simulink model "SingleStreamSSRwithPL"  (R2020a)
settings: Solver=VariableStepAuto  StartTime=0.0  StopTime=inf  RelTol=1e-3
PreLoadFcn:
  | xmcCheckSlxPath(bdroot)
  | SSR4_init
InitFcn:
  | xmcCheckSlxPath(bdroot)
  | SSR4_init;
undefined symbols (not defined in the file): c, FIR_MultiKernel_cin, FIR_MultiKernel_cincout, FIR_MultiKernel_cout, FramesPerVector, S, SHIFT_ACC, SingleStream, T, Taps, ValidDelay, VectorSize, xc7vx485tffg1157
libraries: xbsIndex_r4 x49, ModelComposer x41, simulink x25, dspsrcs4 x1
(part 1 of 3)
settings Model: Creator=oliviert  LastModifiedBy=viswanad

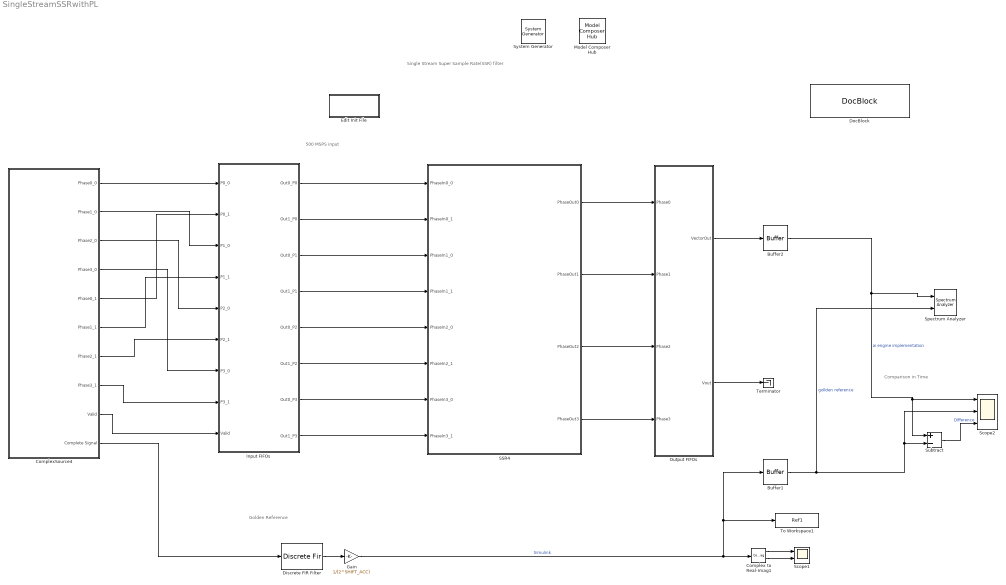
== system SingleStreamSSRwithPL ==
  note: Golden Reference
  note: Single Stream Super Sample Rate(SSR) filter
  note: Comparison in Time
  note: 500 MSPS input
  " System Generator" : xbsIndex_r4/ System Generator  Tag=genX  xilinxfamily=versalaicore  part=xcvc1902  speed=-2MP-e-S  package=vsva2197  synthesis_tool=Vivado  clock_wrapper=Clock Enables  directory=./netlist  proj_type=Vivado  Synth_file=Vivado Synthesis Defaults  Impl_file=Vivado Implementation Defaults  testbench=off  simulink_period=1  sysclk_period=10  dcm_input_clock_period=10  incr_netlist=off  trim_vbits=Everywhere in SubSystem  dbl_ovrd=According to Block Masks  core_generation=According to Block Masks  run_coregen=off  deprecated_control=off  eval_field=0  block_type=sysgen
  Buffer1 : Buffer  N=16  OutputFrames=off
  Buffer2 : Buffer  N=16  OutputFrames=off
  Complex to Real-Imag1 : ComplexToRealImag
  ComplexSource4 : Subsystem  mask{s=0}
      mask prompts: s "Seed"
  Discrete FIR Filter : DiscreteFir  Coefficients=Taps  InputProcessing=Columns as channels (frame based)
  DocBlock : simulink/Model-Wide Utilities/DocBlock  DocumentType=Text  mask(DocBlock){}
      content=|
      | ///////////////////////////////////////////////////////////////////////////
      | // Copyright 2020 Xilinx
      | //
      | // Licensed under the Apache License, Version 2.0 (the "License");
      | // you may not use this file except in compliance with the License.
      | // You may obtain a copy of the License at
      | //
      | // http://www.apache.org/licenses/LICENSE-2.0
      | //
      | // Unless required by applicable law or agreed to in writing, software
      | // distributed under the License is distributed on an "AS IS" BASIS,
      | // WITHOUT WARRANTIES OR CONDITIONS OF ANY KIND, either express or implied.
      | // See the License for the specific language governing permissions and
      | // limitations under the License.
      | ///////////////////////////////////////////////////////////////////////////
      mask Display:
      | xmcDrawBlockIcon();
      | disp(['{\fontsize{10pt}(c) Copyright 2020' ' Xilinx, Inc.}\newline \newline '],'texmode','on');
      | disp('{\fontsize{10pt}Licensed under the Apache License 2.0}','texmode','on');
      | disp('\newline \newline \newline{\fontsize{10pt}Double Click for Copyright Notice}','texmode','on');
  Edit Init File : Subsystem
      settings: OpenFcn=edit('SSR4_init.m');
  Gain : Gain  Gain=1/(2^SHIFT_ACC)
  Input FIFOs : Subsystem
  Model Composer Hub : ModelComposer/Model Composer Hub  CodeGeneration=off  SubsystemName=SSR4  TargetDirectory=./code  ExportType=AI Engines  IpVendor=xilinx.com  IpLibrary=hls  IpVersion=1.0  IpHWLanguage=Verilog  AieCompilerOptions={}  CreateTestbench=on  TestbenchStackSize=10  RunAieSim=on  AieSimTimeout=5000  RunAieSimProfiling=off  LaunchVitisAnalyzer=on  PlotOutput=off  RunX86Sim=off  X86SimTimeout=10  GenHwImage=off  PlatformType=Not Specified  ProjDevice=xc7vx485tffg1157-1  ProjDevicePart=xc7vx485tffg1157-1  SamplePeriod=-1  ClockFrequency=200  DataPathParallelism=1
  Output FIFOs : Subsystem
  SSR4 : Subsystem
  Scope1 : Scope  NumInputPorts=2
  Scope2 : Scope  NumInputPorts=3
  Spectrum Analyzer : SpectrumAnalyzer  NumInputPorts=2
  Subtract : Sum  Inputs=+-
  Terminator : Terminator
  To Workspace1 : ToWorkspace  VariableName=Ref1  SampleTime=-1
      settings: Save2DSignal=2-D array (concatenate along first dimension)
  wires:
  ComplexSource4/10(Complete Signal) -> Discrete FIR Filter/1
  Discrete FIR Filter/1 -> Gain/1
  ComplexSource4/2(Phase1_0) -> Input FIFOs/3(P1_0)
  ComplexSource4/3(Phase2_0) -> Input FIFOs/5(P2_0)
  ComplexSource4/4(Phase3_0) -> Input FIFOs/7(P3_0)
  ComplexSource4/9(Valid) -> Input FIFOs/9(Valid)
  ComplexSource4/5(Phase0_1) -> Input FIFOs/2(P0_1)
  ComplexSource4/6(Phase1_1) -> Input FIFOs/4(P1_1)
  ComplexSource4/7(Phase2_1) -> Input FIFOs/6(P2_1)
  ComplexSource4/8(Phase3_1) -> Input FIFOs/8(P3_1)
  ComplexSource4/1(Phase0_0) -> Input FIFOs/1(P0_0)
  Input FIFOs/1(Out0_P0) -> SSR4/1(PhaseIn0_0)
  Input FIFOs/2(Out1_P0) -> SSR4/2(PhaseIn0_1)
  Input FIFOs/3(Out0_P1) -> SSR4/3(PhaseIn1_0)
  Input FIFOs/4(Out1_P1) -> SSR4/4(PhaseIn1_1)
  Input FIFOs/5(Out0_P2) -> SSR4/5(PhaseIn2_0)
  Input FIFOs/6(Out1_P2) -> SSR4/6(PhaseIn2_1)
  Input FIFOs/7(Out0_P3) -> SSR4/7(PhaseIn3_0)
  Input FIFOs/8(Out1_P3) -> SSR4/8(PhaseIn3_1)
  Subtract/1 -> Scope2/3  "Difference"
  Complex to Real-Imag1/2 -> Scope1/2
  SSR4/1(PhaseOut0) -> Output FIFOs/1(Phase0)
  Complex to Real-Imag1/1 -> Scope1/1
  Gain/1 -> Buffer1/1, To Workspace1/1, Complex to Real-Imag1/1  "Simulink"
  Buffer1/1 -> Spectrum Analyzer/2, Subtract/2, Scope2/2  "gollden reference"
  Output FIFOs/1(VectorOut) -> Buffer2/1
  SSR4/2(PhaseOut1) -> Output FIFOs/2(Phase1)
  SSR4/3(PhaseOut2) -> Output FIFOs/3(Phase2)
  SSR4/4(PhaseOut3) -> Output FIFOs/4(Phase3)
  Buffer2/1 -> Subtract/1, Scope2/1, Spectrum Analyzer/1  "ai engine implementation"
  Output FIFOs/2(Vout) -> Terminator/1

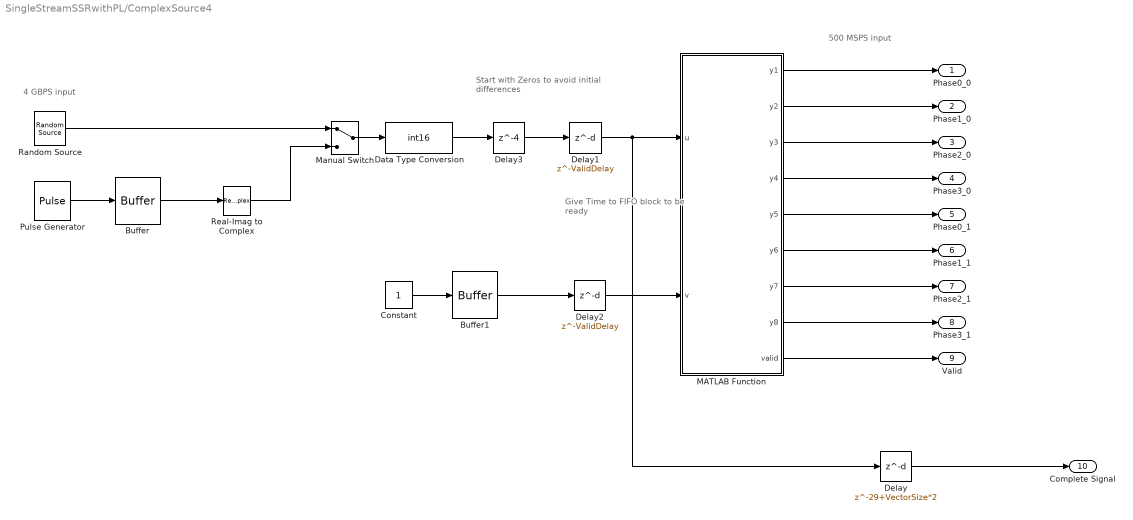
== system SingleStreamSSRwithPL/ComplexSource4 ==
  note: Give Time to
      | FIFO block
      | to be ready
  note: Start with Zeros
      | to avoid
      | initial differences
  note: 4 GBPS input
  note: 500 MSPS input
  Buffer : Buffer  N=VectorSize  OutputFrames=off
  Buffer1 : Buffer  N=FramesPerVector  OutputFrames=off
  Constant : Constant  SampleTime=1
  Data Type Conversion : DataTypeConversion  OutDataTypeStr=int16
  Delay : Delay  DelayLength=29+VectorSize*2  InputProcessing=Columns as channels (frame based)
  Delay1 : Delay  DelayLength=ValidDelay
  Delay2 : Delay  DelayLength=ValidDelay
  Delay3 : Delay  DelayLength=4
  MATLAB Function : MATLAB Function  TreatAsAtomicUnit=on
  Manual Switch : ManualSwitch
  Pulse Generator : DiscretePulseGenerator  Amplitude=20000  Period=32 + 40*5  PhaseDelay=32  SampleTime=1/T
  Random Source : dspsrcs4/Random Source  SrcType=Uniform  NormMethod=Ziggurat  CltLength=12  MinVal=-20000  MaxVal=20000  MeanVal=0  VarVal=1  RepMode=Specify seed  rawSeed=s  IsInherit=off  SampMode=Discrete  SampTime=1/T  SampFrame=VectorSize  DataType=Double  OutComplex=Complex  OutputFrames=off
  Real-Imag to Complex : RealImagToComplex  Input=Real
  Phase0_0 : Outport
  Phase1_0 : Outport  Port=2
  Phase2_0 : Outport  Port=3
  Phase3_0 : Outport  Port=4
  Phase0_1 : Outport  Port=5
  Phase1_1 : Outport  Port=6
  Phase2_1 : Outport  Port=7
  Phase3_1 : Outport  Port=8
  Valid : Outport  Port=9
  Complete Signal : Outport  Port=10
  wires:
  MATLAB Function/1(y1) -> Phase0_0/1
  MATLAB Function/2(y2) -> Phase1_0/1
  MATLAB Function/3(y3) -> Phase2_0/1
  MATLAB Function/4(y4) -> Phase3_0/1
  Real-Imag to Complex/1 -> Manual Switch/2
  Pulse Generator/1 -> Buffer/1
  Delay/1 -> Complete Signal/1
  Buffer/1 -> Real-Imag to Complex/1
  Manual Switch/1 -> Data Type Conversion/1
  MATLAB Function/9(valid) -> Valid/1
  MATLAB Function/8(y8) -> Phase3_1/1
  MATLAB Function/7(y7) -> Phase2_1/1
  MATLAB Function/6(y6) -> Phase1_1/1
  MATLAB Function/5(y5) -> Phase0_1/1
  Random Source/1 -> Manual Switch/1
  Delay1/1 -> Delay/1, MATLAB Function/1(u)
  Delay2/1 -> MATLAB Function/2(v)
  Constant/1 -> Buffer1/1
  Buffer1/1 -> Delay2/1
  Data Type Conversion/1 -> Delay3/1
  Delay3/1 -> Delay1/1

== system SingleStreamSSRwithPL/Edit Init File ==

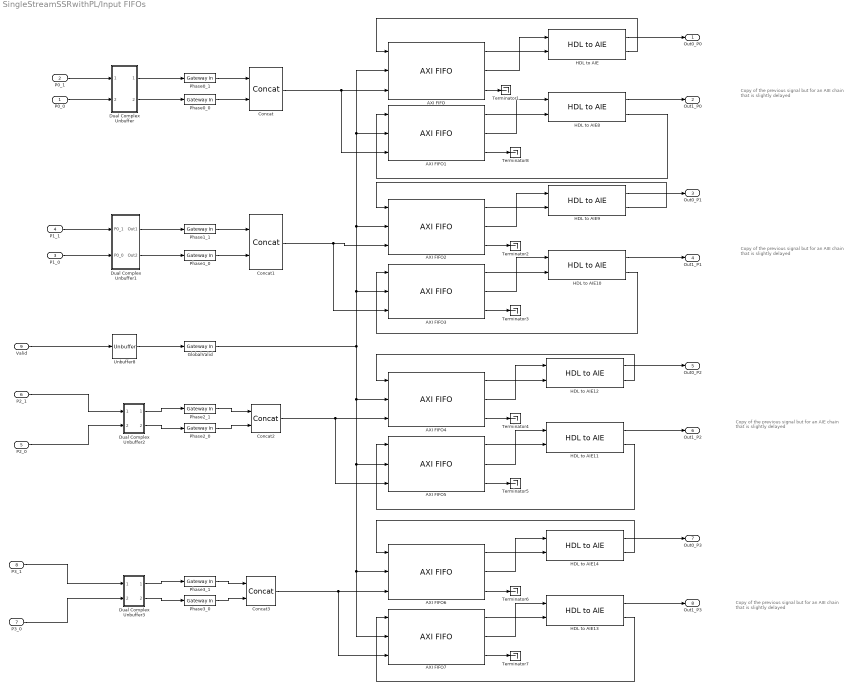
== system SingleStreamSSRwithPL/Input FIFOs ==
  note: Copy of the previous signal
      | but for an AIE chain that is slightly
      | delayed
  note: Copy of the previous signal
      | but for an AIE chain that is slightly
      | delayed
  note: Copy of the previous signal
      | but for an AIE chain that is slightly
      | delayed
  note: Copy of the previous signal
      | but for an AIE chain that is slightly
      | delayed
  P0_0 : Inport
  P0_1 : Inport  Port=2
  P1_0 : Inport  Port=3
  P1_1 : Inport  Port=4
  P2_0 : Inport  Port=5
  P2_1 : Inport  Port=6
  P3_0 : Inport  Port=7
  P3_1 : Inport  Port=8
  Valid : Inport  Port=9
  AXI FIFO{,1..7} (8 alike) : xbsIndex_r4/AXI FIFO  input_depth_axis=512  actual_fifo_depth_label=514  enable_tdata=on  enable_tdest=off  enable_tstrb=off  enable_tready=on  enable_tid=off  enable_tuser=off  enable_tkeep=off  enable_tlast=off  has_aresetn=off  enable_data_counts_axis=off  fifo_implementation_type_axis=Common Clock Block RAM  trim_axipin_name=on  programmable_full_type_axis=Full  full_threshold_assert_value_axis=0  programmable_empty_type_axis=Empty  empty_threshold_assert_value_axis=1022  underflow_flag_axi=0  underflow_sense_axi=Active High  overflow_flag_axi=0  overflow_sense_axi=Active High  simulation_type=fast_sim  block_type=axi_fifo
  Concat{,1..3} (4 alike) : xbsIndex_r4/Concat  num_inputs=2  dbl_ovrd=off  block_type=concat
  Dual Complex Unbuffer : Subsystem
  Dual Complex Unbuffer1 : Subsystem
  Dual Complex Unbuffer2 : Subsystem
  Dual Complex Unbuffer3 : Subsystem
  GlobalValid : xbsIndex_r4/Gateway In  gui_display_data_type=Boolean  arith_type=Boolean  n_bits=16  bin_pt=14  preci_type=Single  exp_width=8  frac_width=24  rows=1  columns=1  quantization="Round  (unbiased: +/- Inf)"  overflow=Saturate  period=1  UseAsADC=off  ADCChannel='1'  interface=None  automatic_assignment=on  address_offset=hex2dec('00')  intf_name=''  intf_description=''  default_value=0  timing_constraint=None  locs_specified=off  LOCs={}  io_standard={}  inherit_from_input=off  hdl_port=on  dbl_ovrd=off  block_type=gatewayin
  HDL to AIE{,8..14} (8 alike) : ModelComposer/HDL to AIE  OutDataType=int16 (c)  OutSampleTime=4/T  SamplesPerFrame=4  TreadySampleTime=1
  Phase0_0 : xbsIndex_r4/Gateway In  gui_display_data_type=Fixed-point  arith_type=Unsigned  n_bits=32  bin_pt=0  preci_type=Single  exp_width=8  frac_width=24  rows=1  columns=1  quantization="Round  (unbiased: +/- Inf)"  overflow=Saturate  period=1  UseAsADC=off  ADCChannel='1'  interface=None  automatic_assignment=on  address_offset=hex2dec('00')  intf_name=''  intf_description=''  default_value=0  timing_constraint=None  locs_specified=off  LOCs={}  io_standard={}  inherit_from_input=off  hdl_port=on  dbl_ovrd=off  block_type=gatewayin
  Phase0_1 : xbsIndex_r4/Gateway In  gui_display_data_type=Fixed-point  arith_type=Unsigned  n_bits=32  bin_pt=0  preci_type=Single  exp_width=8  frac_width=24  rows=1  columns=1  quantization="Round  (unbiased: +/- Inf)"  overflow=Saturate  period=1  UseAsADC=off  ADCChannel='1'  interface=None  automatic_assignment=on  address_offset=hex2dec('00')  intf_name=''  intf_description=''  default_value=0  timing_constraint=None  locs_specified=off  LOCs={}  io_standard={}  inherit_from_input=off  hdl_port=on  dbl_ovrd=off  block_type=gatewayin
  Phase1_0 : xbsIndex_r4/Gateway In  gui_display_data_type=Fixed-point  arith_type=Unsigned  n_bits=32  bin_pt=0  preci_type=Single  exp_width=8  frac_width=24  rows=1  columns=1  quantization="Round  (unbiased: +/- Inf)"  overflow=Saturate  period=1  UseAsADC=off  ADCChannel='1'  interface=None  automatic_assignment=on  address_offset=hex2dec('00')  intf_name=''  intf_description=''  default_value=0  timing_constraint=None  locs_specified=off  LOCs={}  io_standard={}  inherit_from_input=off  hdl_port=on  dbl_ovrd=off  block_type=gatewayin
  Phase1_1 : xbsIndex_r4/Gateway In  gui_display_data_type=Fixed-point  arith_type=Unsigned  n_bits=32  bin_pt=0  preci_type=Single  exp_width=8  frac_width=24  rows=1  columns=1  quantization="Round  (unbiased: +/- Inf)"  overflow=Saturate  period=1  UseAsADC=off  ADCChannel='1'  interface=None  automatic_assignment=on  address_offset=hex2dec('00')  intf_name=''  intf_description=''  default_value=0  timing_constraint=None  locs_specified=off  LOCs={}  io_standard={}  inherit_from_input=off  hdl_port=on  dbl_ovrd=off  block_type=gatewayin
  Phase2_0 : xbsIndex_r4/Gateway In  gui_display_data_type=Fixed-point  arith_type=Unsigned  n_bits=32  bin_pt=0  preci_type=Single  exp_width=8  frac_width=24  rows=1  columns=1  quantization="Round  (unbiased: +/- Inf)"  overflow=Saturate  period=1  UseAsADC=off  ADCChannel='1'  interface=None  automatic_assignment=on  address_offset=hex2dec('00')  intf_name=''  intf_description=''  default_value=0  timing_constraint=None  locs_specified=off  LOCs={}  io_standard={}  inherit_from_input=off  hdl_port=on  dbl_ovrd=off  block_type=gatewayin
  Phase2_1 : xbsIndex_r4/Gateway In  gui_display_data_type=Fixed-point  arith_type=Unsigned  n_bits=32  bin_pt=0  preci_type=Single  exp_width=8  frac_width=24  rows=1  columns=1  quantization="Round  (unbiased: +/- Inf)"  overflow=Saturate  period=1  UseAsADC=off  ADCChannel='1'  interface=None  automatic_assignment=on  address_offset=hex2dec('00')  intf_name=''  intf_description=''  default_value=0  timing_constraint=None  locs_specified=off  LOCs={}  io_standard={}  inherit_from_input=off  hdl_port=on  dbl_ovrd=off  block_type=gatewayin
  Phase3_0 : xbsIndex_r4/Gateway In  gui_display_data_type=Fixed-point  arith_type=Unsigned  n_bits=32  bin_pt=0  preci_type=Single  exp_width=8  frac_width=24  rows=1  columns=1  quantization="Round  (unbiased: +/- Inf)"  overflow=Saturate  period=1  UseAsADC=off  ADCChannel='1'  interface=None  automatic_assignment=on  address_offset=hex2dec('00')  intf_name=''  intf_description=''  default_value=0  timing_constraint=None  locs_specified=off  LOCs={}  io_standard={}  inherit_from_input=off  hdl_port=on  dbl_ovrd=off  block_type=gatewayin
  Phase3_1 : xbsIndex_r4/Gateway In  gui_display_data_type=Fixed-point  arith_type=Unsigned  n_bits=32  bin_pt=0  preci_type=Single  exp_width=8  frac_width=24  rows=1  columns=1  quantization="Round  (unbiased: +/- Inf)"  overflow=Saturate  period=1  UseAsADC=off  ADCChannel='1'  interface=None  automatic_assignment=on  address_offset=hex2dec('00')  intf_name=''  intf_description=''  default_value=0  timing_constraint=None  locs_specified=off  LOCs={}  io_standard={}  inherit_from_input=off  hdl_port=on  dbl_ovrd=off  block_type=gatewayin
  Terminator{1..8} (8 alike) : Terminator
  Unbuffer8 : Unbuffer
  Out0_P0 : Outport
  Out1_P0 : Outport  Port=2
  Out0_P1 : Outport  Port=3
  Out1_P1 : Outport  Port=4
  Out0_P2 : Outport  Port=5
  Out1_P2 : Outport  Port=6
  Out0_P3 : Outport  Port=7
  Out1_P3 : Outport  Port=8
  wires:
  P0_0/1 -> Dual Complex Unbuffer/2(P0_0)
  Valid/1 -> Unbuffer8/1
  GlobalValid/1 -> AXI FIFO4/2, AXI FIFO6/2, AXI FIFO7/2, AXI FIFO5/2, AXI FIFO3/2, AXI FIFO2/2, AXI FIFO1/2, AXI FIFO/2
  Phase2_1/1 -> Concat2/1
  Phase2_0/1 -> Concat2/2
  Phase3_1/1 -> Concat3/1
  Phase3_0/1 -> Concat3/2
  Phase1_0/1 -> Concat1/2
  Phase1_1/1 -> Concat1/1
  Phase0_1/1 -> Concat/1
  Phase0_0/1 -> Concat/2
  Concat/1 -> AXI FIFO1/3, AXI FIFO/3
  AXI FIFO1/3 -> Terminator8/1
  Concat1/1 -> AXI FIFO3/3, AXI FIFO2/3
  AXI FIFO2/3 -> Terminator2/1
  AXI FIFO3/3 -> Terminator3/1
  AXI FIFO5/3 -> Terminator5/1
  AXI FIFO4/3 -> Terminator4/1
  Concat2/1 -> AXI FIFO5/3, AXI FIFO4/3
  AXI FIFO6/3 -> Terminator6/1
  AXI FIFO7/3 -> Terminator7/1
  Concat3/1 -> AXI FIFO7/3, AXI FIFO6/3
  AXI FIFO/1 -> HDL to AIE/2
  AXI FIFO/2 -> HDL to AIE/1
  HDL to AIE/1 -> Out0_P0/1
  AXI FIFO1/1 -> HDL to AIE8/2
  AXI FIFO1/2 -> HDL to AIE8/1
  HDL to AIE8/1 -> Out1_P0/1
  HDL to AIE8/2 -> AXI FIFO1/1
  AXI FIFO2/1 -> HDL to AIE9/2
  AXI FIFO3/1 -> HDL to AIE10/2
  AXI FIFO2/2 -> HDL to AIE9/1
  AXI FIFO3/2 -> HDL to AIE10/1
  HDL to AIE10/2 -> AXI FIFO3/1
  HDL to AIE9/1 -> Out0_P1/1
  HDL to AIE10/1 -> Out1_P1/1
  HDL to AIE9/2 -> AXI FIFO2/1
  AXI FIFO4/1 -> HDL to AIE12/2
  AXI FIFO4/2 -> HDL to AIE12/1
  HDL to AIE12/1 -> Out0_P2/1
  HDL to AIE11/1 -> Out1_P2/1
  HDL to AIE12/2 -> AXI FIFO4/1
  AXI FIFO5/1 -> HDL to AIE11/2
  AXI FIFO5/2 -> HDL to AIE11/1
  HDL to AIE11/2 -> AXI FIFO5/1
  AXI FIFO6/1 -> HDL to AIE14/2
  HDL to AIE14/1 -> Out0_P3/1
  HDL to AIE13/1 -> Out1_P3/1
  AXI FIFO6/2 -> HDL to AIE14/1
  AXI FIFO7/1 -> HDL to AIE13/2
  AXI FIFO7/2 -> HDL to AIE13/1
  HDL to AIE14/2 -> AXI FIFO6/1
  HDL to AIE13/2 -> AXI FIFO7/1
  Unbuffer8/1 -> GlobalValid/1
  Dual Complex Unbuffer/1(Out1) -> Phase0_1/1
  Dual Complex Unbuffer/2(Out2) -> Phase0_0/1
  Dual Complex Unbuffer1/1(Out1) -> Phase1_1/1
  Dual Complex Unbuffer1/2(Out2) -> Phase1_0/1
  P1_1/1 -> Dual Complex Unbuffer1/1(P0_1)
  P1_0/1 -> Dual Complex Unbuffer1/2(P0_0)
  Dual Complex Unbuffer2/1(Out1) -> Phase2_1/1
  Dual Complex Unbuffer2/2(Out2) -> Phase2_0/1
  P2_1/1 -> Dual Complex Unbuffer2/1(P0_1)
  P2_0/1 -> Dual Complex Unbuffer2/2(P0_0)
  Dual Complex Unbuffer3/1(Out1) -> Phase3_1/1
  Dual Complex Unbuffer3/2(Out2) -> Phase3_0/1
  P3_1/1 -> Dual Complex Unbuffer3/1(P0_1)
  P3_0/1 -> Dual Complex Unbuffer3/2(P0_0)
  P0_1/1 -> Dual Complex Unbuffer/1(P0_1)
  HDL to AIE/2 -> AXI FIFO/1
  AXI FIFO/3 -> Terminator1/1

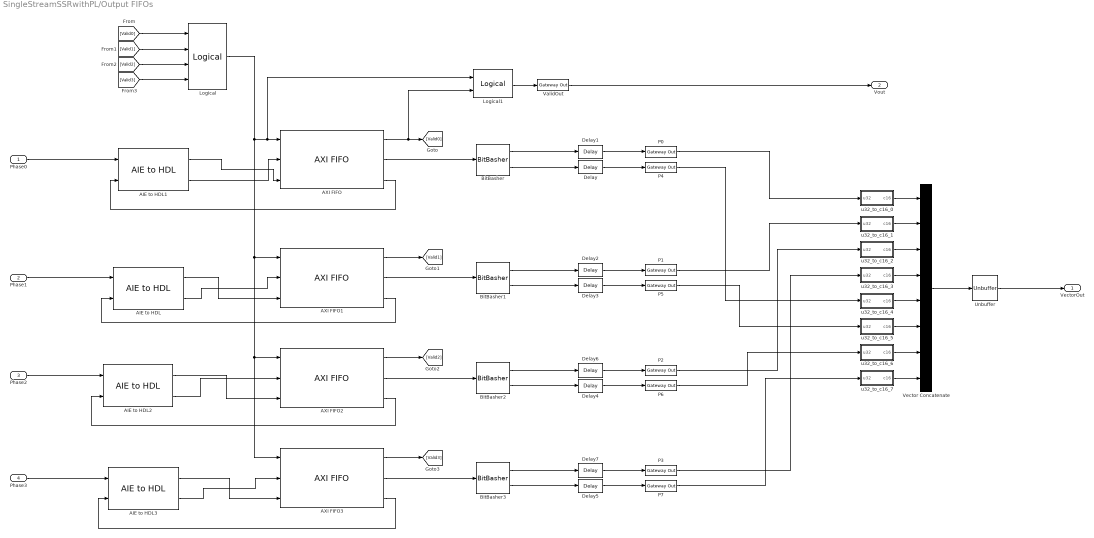
== system SingleStreamSSRwithPL/Output FIFOs ==
  Phase0 : Inport
  Phase1 : Inport  Port=2
  Phase2 : Inport  Port=3
  Phase3 : Inport  Port=4
  AIE to HDL{,1..3} (4 alike) : ModelComposer/AIE to HDL  OutDataType=ufix64  OutSampleTime=1
  AXI FIFO{,1..3} (4 alike) : xbsIndex_r4/AXI FIFO  input_depth_axis=512  actual_fifo_depth_label=514  enable_tdata=on  enable_tdest=off  enable_tstrb=off  enable_tready=on  enable_tid=off  enable_tuser=off  enable_tkeep=off  enable_tlast=off  has_aresetn=off  enable_data_counts_axis=off  fifo_implementation_type_axis=Common Clock Block RAM  trim_axipin_name=on  programmable_full_type_axis=Full  full_threshold_assert_value_axis=0  programmable_empty_type_axis=Empty  empty_threshold_assert_value_axis=1022  underflow_flag_axi=0  underflow_sense_axi=Active High  overflow_flag_axi=0  overflow_sense_axi=Active High  simulation_type=fast_sim  block_type=axi_fifo
  BitBasher : xbsIndex_r4/BitBasher  bitexpr=|  display_expr=off  sr_1=lo  arith_type1=Unsigned  bin_pt1=0  sr_2=hi  arith_type2=Unsigned  bin_pt2=0  sr_3=3  arith_type3=Unsigned  bin_pt3=0  sr_4=4  arith_type4=Unsigned  bin_pt4=0  dbl_ovrd=off  block_type=bitbasher
      | lo={in[31:0]}
      | hi={in[63:32]}
  BitBasher1 : xbsIndex_r4/BitBasher  bitexpr=|  display_expr=off  sr_1=lo  arith_type1=Unsigned  bin_pt1=0  sr_2=hi  arith_type2=Unsigned  bin_pt2=0  sr_3=3  arith_type3=Unsigned  bin_pt3=0  sr_4=4  arith_type4=Unsigned  bin_pt4=0  dbl_ovrd=off  block_type=bitbasher
      | lo={in[31:0]}
      | hi={in[63:32]}
  BitBasher2 : xbsIndex_r4/BitBasher  bitexpr=|  display_expr=off  sr_1=lo  arith_type1=Unsigned  bin_pt1=0  sr_2=hi  arith_type2=Unsigned  bin_pt2=0  sr_3=3  arith_type3=Unsigned  bin_pt3=0  sr_4=4  arith_type4=Unsigned  bin_pt4=0  dbl_ovrd=off  block_type=bitbasher
      | lo={in[31:0]}
      | hi={in[63:32]}
  BitBasher3 : xbsIndex_r4/BitBasher  bitexpr=|  display_expr=off  sr_1=lo  arith_type1=Unsigned  bin_pt1=0  sr_2=hi  arith_type2=Unsigned  bin_pt2=0  sr_3=3  arith_type3=Unsigned  bin_pt3=0  sr_4=4  arith_type4=Unsigned  bin_pt4=0  dbl_ovrd=off  block_type=bitbasher
      | lo={in[31:0]}
      | hi={in[63:32]}
  Delay{,1..7} (8 alike) : xbsIndex_r4/Delay  rst=off  infoeditControl=Selection of Reset will increase slice count due to use of real FFs and instead of SRLs  en=off  latency=1  reg_retiming=off  dbl_ovrd=off  block_type=delay
  Logical : xbsIndex_r4/Logical  logical_function=AND  inputs=4  en=off  latency=0  precision=Full  arith_type=Unsigned  n_bits=16  bin_pt=0  align_bp=on  dbl_ovrd=off  block_type=logical
  Logical1 : xbsIndex_r4/Logical  logical_function=AND  inputs=2  en=off  latency=1  precision=Full  arith_type=Unsigned  n_bits=16  bin_pt=0  align_bp=on  dbl_ovrd=off  block_type=logical
  P{0..7} (8 alike) : xbsIndex_r4/Gateway Out  inherit_from_input=on  hdl_port=on  rows=1  columns=1  UseAsDAC=off  DACChannel='1'  interface=None  automatic_assignment=on  address_offset=hex2dec('00')  intf_name=''  intf_description=''  timing_constraint=None  locs_specified=off  LOCs={}  io_standard={}  block_type=gatewayout
  Unbuffer : Unbuffer
  ValidOut : xbsIndex_r4/Gateway Out  inherit_from_input=off  hdl_port=on  rows=1  columns=1  UseAsDAC=off  DACChannel='1'  interface=None  automatic_assignment=on  address_offset=hex2dec('00')  intf_name=''  intf_description=''  timing_constraint=None  locs_specified=off  LOCs={}  io_standard={}  block_type=gatewayout
  Vector Concatenate : Concatenate  NumInputs=8
  u32_to_c16_0 : Subsystem
  u32_to_c16_1 : Subsystem
  u32_to_c16_2 : Subsystem
  u32_to_c16_3 : Subsystem
  u32_to_c16_4 : Subsystem
  u32_to_c16_5 : Subsystem
  u32_to_c16_6 : Subsystem
  u32_to_c16_7 : Subsystem
  VectorOut : Outport
  Vout : Outport  Port=2
  wires:
  Phase0/1 -> AIE to HDL1/1
  AXI FIFO/3 -> AIE to HDL1/2
  AXI FIFO1/3 -> AIE to HDL/2
  Phase1/1 -> AIE to HDL/1
  Phase2/1 -> AIE to HDL2/1
  AXI FIFO2/3 -> AIE to HDL2/2
  AXI FIFO3/3 -> AIE to HDL3/2
  Phase3/1 -> AIE to HDL3/1
  Logical/1 -> Logical1/1, AXI FIFO/1, AXI FIFO1/1, AXI FIFO2/1, AXI FIFO3/1
  AXI FIFO/1 -> Logical1/2, [Valid0]
  AXI FIFO1/1 -> [Valid1]
  AXI FIFO2/1 -> [Valid2]
  AXI FIFO3/1 -> [Valid3]
  [Valid0] -> Logical/1
  [Valid1] -> Logical/2
  [Valid2] -> Logical/3
  [Valid3] -> Logical/4
  AXI FIFO/2 -> BitBasher/1
  AXI FIFO1/2 -> BitBasher1/1
  AXI FIFO2/2 -> BitBasher2/1
  AXI FIFO3/2 -> BitBasher3/1
  BitBasher/2 -> Delay/1
  BitBasher1/2 -> Delay3/1
  BitBasher2/2 -> Delay4/1
  BitBasher3/2 -> Delay5/1
  Logical1/1 -> ValidOut/1
  Delay/1 -> P4/1
  BitBasher/1 -> Delay1/1
  Delay1/1 -> P0/1
  Delay3/1 -> P5/1
  BitBasher1/1 -> Delay2/1
  Delay2/1 -> P1/1
  Delay4/1 -> P6/1
  Delay5/1 -> P7/1
  BitBasher2/1 -> Delay6/1
  Delay6/1 -> P2/1
  BitBasher3/1 -> Delay7/1
  Delay7/1 -> P3/1
  P1/1 -> u32_to_c16_1/1(u32)
  P0/1 -> u32_to_c16_0/1(u32)
  P2/1 -> u32_to_c16_2/1(u32)
  P3/1 -> u32_to_c16_3/1(u32)
  P6/1 -> u32_to_c16_6/1(u32)
  P5/1 -> u32_to_c16_5/1(u32)
  P7/1 -> u32_to_c16_7/1(u32)
  P4/1 -> u32_to_c16_4/1(u32)
  Vector Concatenate/1 -> Unbuffer/1
  ValidOut/1 -> Vout/1
  AIE to HDL1/1 -> AXI FIFO/3
  AIE to HDL/1 -> AXI FIFO1/3
  AIE to HDL/2 -> AXI FIFO1/2
  AIE to HDL2/1 -> AXI FIFO2/3
  AIE to HDL2/2 -> AXI FIFO2/2
  AIE to HDL3/1 -> AXI FIFO3/3
  AIE to HDL3/2 -> AXI FIFO3/2
  u32_to_c16_0/1(c16) -> Vector Concatenate/1
  u32_to_c16_1/1(c16) -> Vector Concatenate/2
  u32_to_c16_2/1(c16) -> Vector Concatenate/3
  u32_to_c16_3/1(c16) -> Vector Concatenate/4
  u32_to_c16_4/1(c16) -> Vector Concatenate/5
  u32_to_c16_5/1(c16) -> Vector Concatenate/6
  u32_to_c16_6/1(c16) -> Vector Concatenate/7
  u32_to_c16_7/1(c16) -> Vector Concatenate/8
  Unbuffer/1 -> VectorOut/1
  AIE to HDL1/2 -> AXI FIFO/2
